simulink subsystem "dz1_model"  (R2023a)
settings: Solver=VariableStepAuto  StartTime=0.0  StopTime=10.0  RelTol=1e-3
settings Model: Creator=diontep  LastModifiedBy=diontep

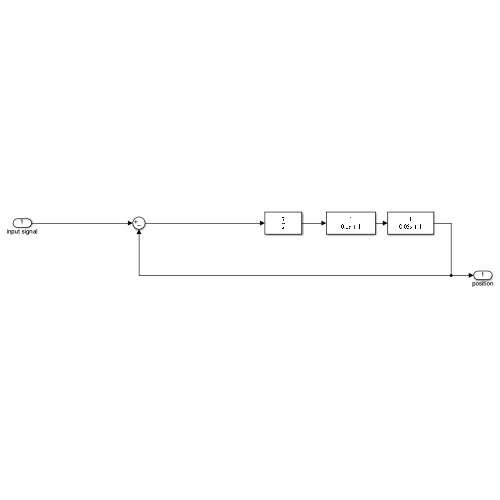
[thumbnail: Simulink's stored preview of the top-level diagram]
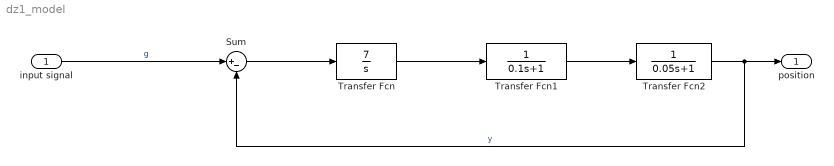
== system dz1_model ==
  input signal : Inport
  Sum : Sum  Inputs=|+-
  Transfer Fcn : TransferFcn  Numerator=[7]  Denominator=[1 0]
  Transfer Fcn1 : TransferFcn  Denominator=[0.1 1]
  Transfer Fcn2 : TransferFcn  Denominator=[0.05 1]
  position : Outport
  wires:
  input signal/1 -> Sum/1  "g"
  Transfer Fcn1/1 -> Transfer Fcn2/1
  Transfer Fcn/1 -> Transfer Fcn1/1
  Transfer Fcn2/1 -> position/1, Sum/2  "y"
  Sum/1 -> Transfer Fcn/1
